simulink model "Frequency_converter"  (R2023b)
settings: Solver=ode45  StartTime=0.0  StopTime=0.1  RelTol=1e-3
libraries: spsDiodeLib x12, spsIdealSwitchLib x6, spsTriangleGeneratorLib x3, spsCurrentMeasurementLib x2, spsVoltageMeasurementLib x2, spsGroundLib x1, spsThreePhaseProgrammableVoltageSourceLib x1, spsThreePhaseSeriesRLCBranchLib x1, spsVariableCapacitorLib x1, spspowerguiLib x1
settings Model: Creator=LX  LastModifiedBy=Ngsanchong
settings DataIOCC: ReturnWorkspaceOutputs=off

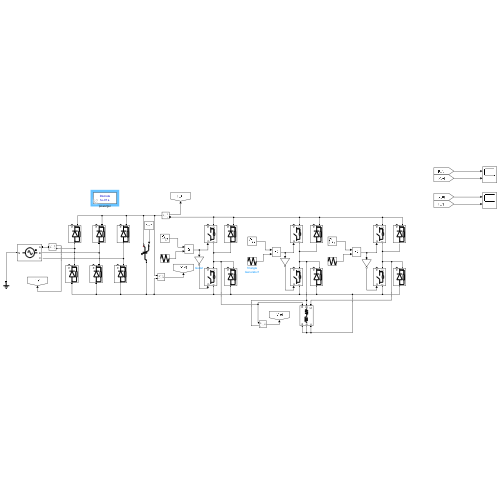
[thumbnail: Simulink's stored preview of the top-level diagram]
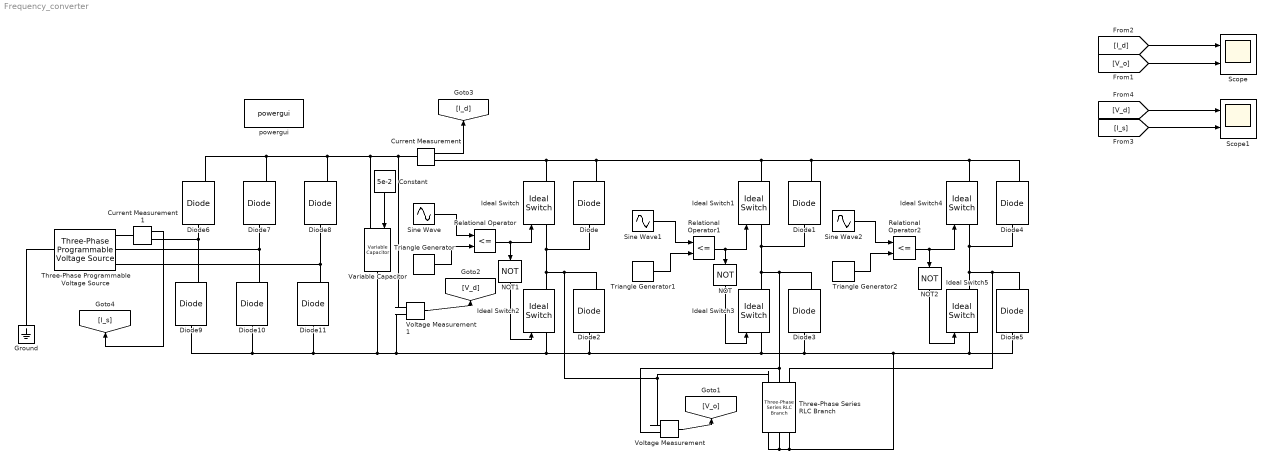
== system Frequency_converter ==
  Constant : Constant  Value=5e-2
  Current Measurement : spsCurrentMeasurementLib/Current Measurement  PhasorSimulation=off  OutputType=Complex  PSBequivalent=0
  Current Measurement1 : spsCurrentMeasurementLib/Current Measurement  PhasorSimulation=off  OutputType=Complex  PSBequivalent=0
  Diode{,1..11} (12 alike) : spsDiodeLib/Diode  Ron=0.001  Lon=0  Vf=0.8  IC=0  UseSnubber=0  Rs=500  Cs=250e-9  Measurements=on
  Ground : spsGroundLib/Ground  LConnTagsString=a
  Ideal Switch{,1..5} (6 alike) : spsIdealSwitchLib/Ideal Switch  Ron=1e-9  Lon=0  IC=0  Rs=1e5  Cs=inf  Measurements=on
  NOT : Logic  Operator=NOT  IconShape=distinctive  AllPortsSameDT=off  OutDataTypeStr=boolean
  NOT1 : Logic  Operator=NOT  IconShape=distinctive  AllPortsSameDT=off  OutDataTypeStr=boolean
  NOT2 : Logic  Operator=NOT  IconShape=distinctive  AllPortsSameDT=off  OutDataTypeStr=boolean
  Relational Operator : RelationalOperator  Operator=<=  OutDataTypeStr=boolean  RndMeth=Simplest  InputSameDT=off
  Relational Operator1 : RelationalOperator  Operator=<=  OutDataTypeStr=boolean  RndMeth=Simplest  InputSameDT=off
  Relational Operator2 : RelationalOperator  Operator=<=  OutDataTypeStr=boolean  RndMeth=Simplest  InputSameDT=off
  Scope : Scope  NumInputPorts=2
  Scope1 : Scope  NumInputPorts=2
  Sine Wave : Sin  Amplitude=0.8  Frequency=2*pi*50  SampleTime=0
  Sine Wave1 : Sin  Amplitude=0.8  Frequency=2*pi*50  Phase=-2*pi/3  SampleTime=0
  Sine Wave2 : Sin  Amplitude=0.8  Frequency=2*pi*50  Phase=2*pi/3  SampleTime=0
  Three-Phase Programmable Voltage Source : spsThreePhaseProgrammableVoltageSourceLib/Three-Phase Programmable Voltage Source  PositiveSequence=[(380)*1 0 50]  VariationEntity=None  VariationType=Table of time-amplitude pairs  VariationTypeAlt=Step  VariationStep=0.5  VariationRate=10  VariationMagnitude=0.3  VariationFrequency=2  VariationTiming=[1 2]  VariationPhaseA=off  Amplitudes=[1 0.8 1.2 1.0]  TimeValues=[0 0.1 0.15 0.2]  HarmonicGeneration=off  HarmonicA=[3 0.2 -25 0]  HarmonicB=[2 0.15 35 2]  Timing="[0.05  3]"  BusType=swing  Pref=0  Qref=0  Qmin=-Inf  Qmax=Inf
  Three-Phase Series RLC Branch : spsThreePhaseSeriesRLCBranchLib/Three-Phase Series RLC Branch  LConnTagsString=A|B|C  RConnTagsString=A|B|C  BranchType=RL  Resistance=5  Inductance=5e-3  Capacitance=1e-6  Measurements=None
  Triangle Generator : spsTriangleGeneratorLib/Triangle Generator  Freq=1950  Phase=90  Ts=0
  Triangle Generator1 : spsTriangleGeneratorLib/Triangle Generator  Freq=1950  Phase=90  Ts=0
  Triangle Generator2 : spsTriangleGeneratorLib/Triangle Generator  Freq=1950  Phase=90  Ts=0
  Variable Capacitor : spsVariableCapacitorLib/Variable Capacitor  methode=Backward Euler  Cabsmin=1e-9  Initialize=off  vC0=0  C0=1e-6  iC0=-7.0395e-18
      settings: LibrarySourceBlock=sps_lib/Passives/Variable Capacitor
  Voltage Measurement : spsVoltageMeasurementLib/Voltage Measurement  PhasorSimulation=off  OutputType=Complex  PSBequivalent=0
  Voltage Measurement1 : spsVoltageMeasurementLib/Voltage Measurement  PhasorSimulation=off  OutputType=Complex  PSBequivalent=0
  powergui : spspowerguiLib/powergui  Priority=1  SimulationMode=Discrete  SampleTime=1e-7  frequency=60  Iterations=50  frequencyindice=0  Pbase=100e6  ErrMax=1e-4  UnitsV=kV  UnitsW=MW  buscounter=0  FunctionMessages=off  echomessages=off  EnableUseOfTLC=off  CurrentSourceSwitches=off  DisableSnubberDevices=off  DisableRonSwitches=off  DisableVfSwitches=off  DisplayEquations=off  AutomaticDiscreteSolvers=off  SolverType=Tustin/Backward Euler (TBE)  Interpol=off  ExternalGateDelay=off  methode=off  Ts=100  x0status=blocks  SPID=on  SwTol=0  HookPort=off  NonlinearTolerance=1e-4  nMaxIteration=100  ContinueOnMaxIteration=off  RestoreLinks=warning  ResistiveCurrentMeasurement=off  Frange=[0:2:500]  Ylog=off  Xlog=on  ShowGrid=off  save=off  variable=ZData  structure=0  ZoomFFT=off  StartTime=0.0  cycles=1  DisplayStyle=1  fundamental=60  FreqAxis=off  MaxFrequency=1000  frequencyindicesteady=1  RmsSteady=1  display=off
  wires:
  Sine Wave/1 -> Relational Operator/1
  Triangle Generator/1 -> Relational Operator/2
  Relational Operator/1 -> NOT1/1, Ideal Switch/1
  Current Measurement/1 -> [I_d]
  Voltage Measurement/1 -> [V_o]
  Triangle Generator1/1 -> Relational Operator1/2
  Sine Wave1/1 -> Relational Operator1/1
  Relational Operator1/1 -> NOT/1, Ideal Switch1/1
  NOT/1 -> Ideal Switch3/1
  NOT1/1 -> Ideal Switch2/1
  Triangle Generator2/1 -> Relational Operator2/2
  Sine Wave2/1 -> Relational Operator2/1
  NOT2/1 -> Ideal Switch5/1
  Relational Operator2/1 -> Ideal Switch4/1, NOT2/1
  Constant/1 -> Variable Capacitor/1
  Voltage Measurement1/1 -> [V_d]
  Current Measurement1/1 -> [I_s]
  [V_o] -> Scope/2
  [I_d] -> Scope/1
  [I_s] -> Scope1/2
  [V_d] -> Scope1/1
  connections:
  Ideal Switch4/RConn1 -- Ideal Switch/RConn1 -- Current Measurement/RConn1 -- Diode/RConn1 -- Ideal Switch1/RConn1 -- Diode1/RConn1 -- Diode4/RConn1
  Ideal Switch2/RConn1 -- Voltage Measurement/LConn1 -- Three-Phase Series RLC Branch/LConn1 -- Diode2/RConn1 -- Ideal Switch/LConn1 -- Diode/LConn1
  Ideal Switch3/RConn1 -- Ideal Switch1/LConn1 -- Diode1/LConn1 -- Three-Phase Series RLC Branch/LConn2 -- Voltage Measurement/LConn2 -- Diode3/RConn1
  Ideal Switch5/LConn1 -- Three-Phase Series RLC Branch/RConn1 -- Three-Phase Series RLC Branch/RConn2 -- Three-Phase Series RLC Branch/RConn3 -- Voltage Measurement1/LConn2 -- Variable Capacitor/RConn1 -- Diode9/LConn1 -- Diode10/LConn1 -- Diode11/LConn1 -- Ideal Switch2/LConn1 -- Diode2/LConn1 -- Ideal Switch3/LConn1 -- Diode3/LConn1 -- Diode5/LConn1
  Diode4/LConn1 -- Ideal Switch5/RConn1 -- Three-Phase Series RLC Branch/LConn3 -- Diode5/RConn1 -- Ideal Switch4/LConn1
  Diode9/RConn1 -- Diode6/LConn1 -- Current Measurement1/RConn1
  Diode10/RConn1 -- Three-Phase Programmable Voltage Source/RConn2 -- Diode7/LConn1
  Diode11/RConn1 -- Three-Phase Programmable Voltage Source/RConn3 -- Diode8/LConn1
  Diode7/RConn1 -- Diode6/RConn1 -- Voltage Measurement1/LConn1 -- Current Measurement/LConn1 -- Variable Capacitor/LConn1 -- Diode8/RConn1
  Ground/LConn1 -- Three-Phase Programmable Voltage Source/LConn1
  Current Measurement1/LConn1 -- Three-Phase Programmable Voltage Source/RConn1
